simulink model "Aufgabe2"  (R2016a)
settings: Solver=ode45  StartTime=0.0  StopTime=2.2  RelTol=1e-3
libraries: simulink x2
settings Model: Creator=Bornitz  LastModifiedBy=Bornitz
settings DataIOCC: LimitDataPoints=on  SaveFormat=Array
settings DebuggingCC: StateNameClashWarn=warning  StrictBusMsg=ErrorOnBusTreatedAsVector
settings HardwareCC: ProdBitPerPointer=32  ProdLargestAtomicFloat=None  ProdIntDivRoundTo=Undefined  ProdEndianess=Unspecified  ProdWordSize=32  ProdHWDeviceType=32-bit Generic
settings ModelReferenceCC: PropagateSignalLabelsOutOfModel=off
settings ConfigComp: CovModelRefEnable=Off

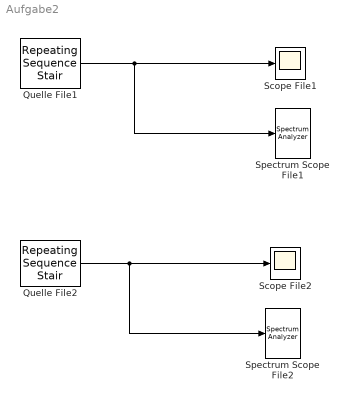
== system Aufgabe2 ==
  Quelle File1 : simulink/Sources/Repeating Sequence Stair  OutValues=us1  tsamp=1/32000  OutMin=[]  OutMax=[]  OutDataTypeStr=double  OutputDataTypeScalingMode=double  OutDataType=fixdt(0,8)  ConRadixGroup=Best Precision: Vector-wise  OutScaling=2^-12
  Quelle File2 : simulink/Sources/Repeating Sequence Stair  OutValues=us2  tsamp=1/80000  OutMin=[]  OutMax=[]  OutDataTypeStr=double  OutputDataTypeScalingMode=double  OutDataType=fixdt(0,8)  ConRadixGroup=Best Precision: Vector-wise  OutScaling=2^-12
  Scope File1 : Scope
  Scope File2 : Scope
  Spectrum Scope File1 : SpectrumAnalyzer
  Spectrum Scope File2 : SpectrumAnalyzer
  wires:
  Quelle File2/1 -> Spectrum Scope File2/1, Scope File2/1
  Quelle File1/1 -> Spectrum Scope File1/1, Scope File1/1
